simulink model "lukenmia_model"  (R2024a)
settings: Solver=VariableStepAuto  StartTime=0.0  StopTime=20  RelTol=1e-3
settings Model: Creator=samad  LastModifiedBy=samad

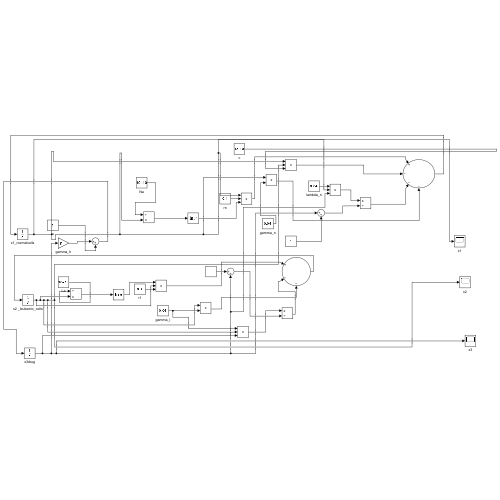
[thumbnail: Simulink's stored preview of the top-level diagram]
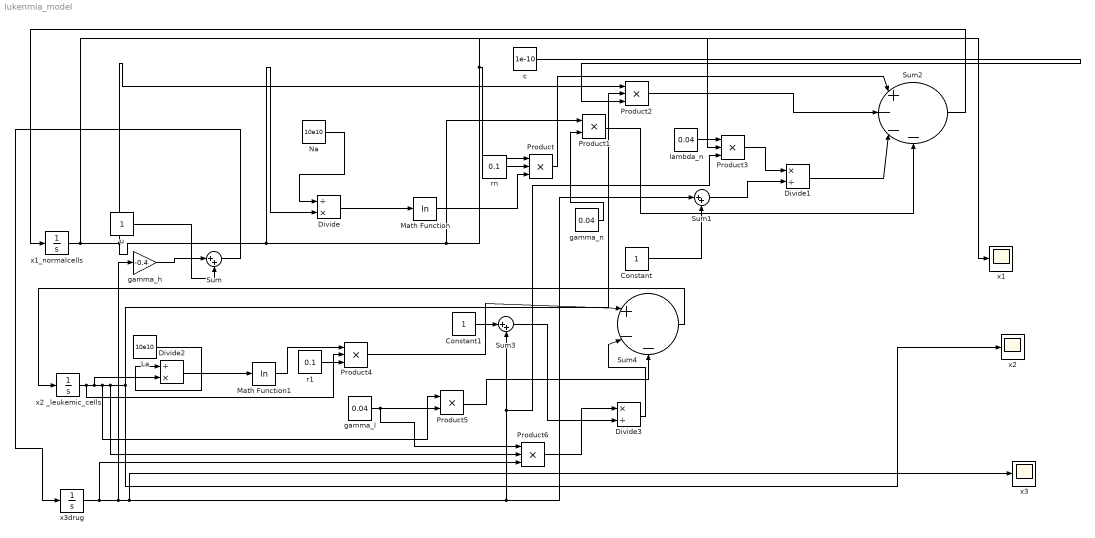
== system lukenmia_model ==
  Constant : Constant
  Constant1 : Constant
  Divide : Product  Inputs=/*
  Divide1 : Product  Inputs=*/
  Divide2 : Product  Inputs=/*
  Divide3 : Product  Inputs=*/
  La : Constant  Value=10e10
  Math Function : Math  Operator=log
  Math Function1 : Math  Operator=log
  Na : Constant  Value=10e10
  Product{,2..4,6} (5 alike) : Product  Inputs=3
  Product1 : Product
  Product5 : Product
  Sum : Sum  Inputs=|++
  Sum1 : Sum  Inputs=|++
  Sum2 : Sum  Inputs=|+---
  Sum3 : Sum  Inputs=|++
  Sum4 : Sum  Inputs=|+--
  c : Constant  Value=1e-10
  gamma_h : Gain  Gain=-0.4
  gamma_l : Constant  Value=0.04
  gamma_n : Constant  Value=0.04
  lambda_n : Constant  Value=0.04
  r1 : Constant  Value=0.1
  rn : Constant  Value=0.1
  u : Constant
  x1 : Scope
  x1_normalcells : Integrator  InitialCondition=10e8
  x2 : Scope
  x2 _leukemic_cells : Integrator  InitialCondition=1.8e8
  x3 : Scope
  x3drug : Integrator
  wires:
  u/1 -> Sum/2
  Sum/1 -> x3drug/1
  Na/1 -> Divide/1
  x1_normalcells/1 -> x1/1, Product3/2, Product/1, Product1/1, Divide/2, Product2/1
  Divide/1 -> Math Function/1
  rn/1 -> Product/2
  Math Function/1 -> Product/3
  gamma_n/1 -> Product1/2
  x2 _leukemic_cells/1 -> Product4/2, Divide2/2, Product5/1, Product6/2, x2/1, Product2/2
  c/1 -> Product2/3
  x3drug/1 -> Product6/3, Sum1/1, Product3/3, Sum3/2, x3/1, gamma_h/1
  Constant/1 -> Sum1/2
  lambda_n/1 -> Product3/1
  Product3/1 -> Divide1/1
  Sum1/1 -> Divide1/2
  Product/1 -> Sum2/1
  Product2/1 -> Sum2/2
  Divide1/1 -> Sum2/3
  Product1/1 -> Sum2/4
  Sum2/1 -> x1_normalcells/1
  La/1 -> Divide2/1
  Divide2/1 -> Math Function1/1
  Math Function1/1 -> Product4/1
  r1/1 -> Product4/3
  gamma_l/1 -> Product6/1, Product5/2
  Constant1/1 -> Sum3/1
  Product6/1 -> Divide3/1
  Sum3/1 -> Divide3/2
  gamma_h/1 -> Sum/1
  Product4/1 -> Sum4/1
  Divide3/1 -> Sum4/2
  Product5/1 -> Sum4/3
  Sum4/1 -> x2 _leukemic_cells/1
